simulink model "cps_slow_network_v2"  (R2012b)
settings: Solver=FixedStepDiscrete  StartTime=0.0  StopTime=8.5  RelTol=20e-5
model workspace (MAT data in the model file):
  ini_block_hpos = -0.4
  ini_block_vpos = 0.11
  ini_nozzle_vpos = 0.3
settings Model: Creator=pmosterm  LastModifiedBy=pmosterm
settings SolverCC: ZcThreshold=2e-5  MaxConsecutiveZCs=20  EnableConcurrentExecution=on  ConcurrentTasks=on  ZeroCrossAlgorithm=Adaptive  SolverResetMethod=Robust
settings DataIOCC: SignalLoggingSaveFormat=ModelDataLogs
settings OptimizationCC: InlineParams=on
settings DebuggingCC: ReadBeforeWriteMsg=DisableAll  WriteAfterWriteMsg=DisableAll  WriteAfterReadMsg=DisableAll  AlgebraicLoopMsg=error  UnderspecifiedInitializationDetection=Simplified  FcnCallInpInsideContextMsg=EnableAllAsWarning  ModelReferenceExtraNoncontSigs=warning
settings ModelReferenceCC: ModelReferenceNumInstancesAllowed=Single
settings GRTTargetCC: CombineOutputUpdateFcns=off  GRTInterface=on
settings ConfigurationSet: Description=SimMechanics 2G

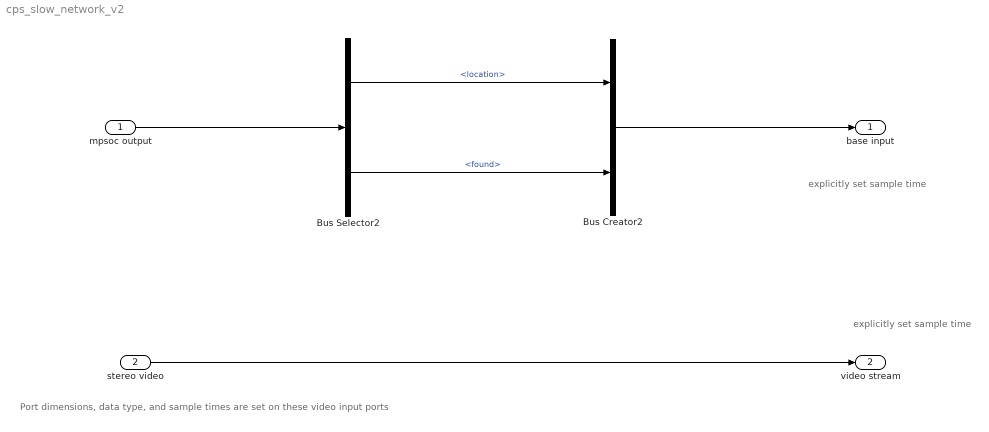
== system cps_slow_network_v2 ==
  note: explicitly set
      | sample time
  note: Port dimensions, data type, and sample times are
      | set on these video input ports
  note: explicitly set
      | sample time
  mpsoc output : Inport  OutDataTypeStr=Bus: slBusStereoOps
  stereo video : Inport  Port=2  OutDataTypeStr=uint8  PortDimensions=[400 240 6]  SampleTime=0.1
  Bus Creator2 : BusCreator  Inputs=2
  Bus Selector2 : BusSelector  OutputSignals=location,found
  base input : Outport  OutDataTypeStr=Bus: slBusStereoOps  SampleTime=0.1  BusOutputAsStruct=on
  video stream : Outport  Port=2  SampleTime=0.1
  wires:
  Bus Selector2/2 -> Bus Creator2/2  "<found>"
  Bus Selector2/1 -> Bus Creator2/1  "<location>"
  mpsoc output/1 -> Bus Selector2/1
  Bus Creator2/1 -> base input/1
  stereo video/1 -> video stream/1
